simulink model "MBSE_Project_SunRoof"  (R2020b)
settings: Solver=VariableStepAuto  StartTime=0.0  StopTime=inf  RelTol=1e-3
settings Model: Creator=99003747  LastModifiedBy=99003747

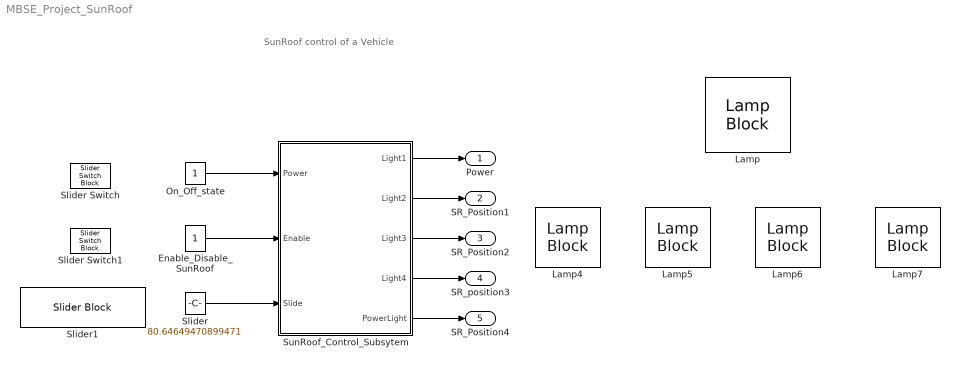
== system MBSE_Project_SunRoof ==
  note: SunRoof control of a Vehicle
  Enable_Disable_SunRoof : Constant
  Lamp{,4..7} (5 alike) : LampBlock
  On_Off_state : Constant
  Slider : Constant  Value=80.64649470899471
  Slider Switch : SliderSwitchBlock
      settings: Values={{'Off', 'On'}, [0 1]}
  Slider Switch1 : SliderSwitchBlock
      settings: Values={{'Off', 'On'}, [0 1]}
  Slider1 : SliderBlock
  SunRoof_Control_Subsytem : Subsystem
      mask Display: image('C:\Users\99003747\Desktop\sunroof.jfif')
  Power : Outport
  SR_Position1 : Outport  Port=2
  SR_Position2 : Outport  Port=3
  SR_position3 : Outport  Port=4
  SR_Position4 : Outport  Port=5
  wires:
  On_Off_state/1 -> SunRoof_Control_Subsytem/1(Power)
  Enable_Disable_SunRoof/1 -> SunRoof_Control_Subsytem/2(Enable)
  Slider/1 -> SunRoof_Control_Subsytem/3(Slide)
  SunRoof_Control_Subsytem/1(Light1) -> Power/1
  SunRoof_Control_Subsytem/2(Light2) -> SR_Position1/1
  SunRoof_Control_Subsytem/3(Light3) -> SR_Position2/1
  SunRoof_Control_Subsytem/4(Light4) -> SR_position3/1
  SunRoof_Control_Subsytem/5(PowerLight) -> SR_Position4/1

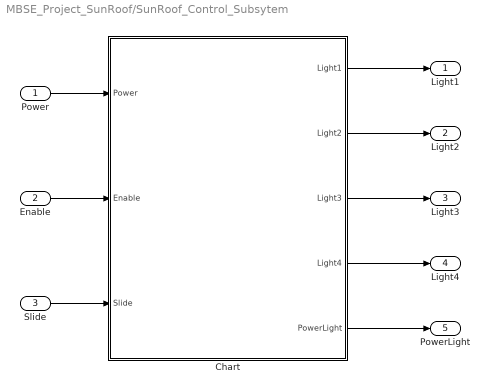
== system MBSE_Project_SunRoof/SunRoof_Control_Subsytem ==
  Power : Inport
  Enable : Inport  Port=2
  Slide : Inport  Port=3
  Chart : Stateflow chart  TreatAsAtomicUnit=on
  Light1 : Outport
  Light2 : Outport  Port=2
  Light3 : Outport  Port=3
  Light4 : Outport  Port=4
  PowerLight : Outport  Port=5
  wires:
  Slide/1 -> Chart/3(Slide)
  Chart/3(Light3) -> Light3/1
  Chart/1(Light1) -> Light1/1
  Chart/2(Light2) -> Light2/1
  Enable/1 -> Chart/2(Enable)
  Power/1 -> Chart/1(Power)
  Chart/4(Light4) -> Light4/1
  Chart/5(PowerLight) -> PowerLight/1

== stateflow chart MBSE_Project_SunRoof/SunRoof_Control_Subsytem/Chart ==
  state PowerOff
    entry:
    PowerLight=0;
    Light1=0;
    Light2=0;
    Light3=0;
    Light4=0;
  state PowerOn
    entry:
    PowerLight=1;
    Light1=0;
    Light2=0;
    Light3=0;
    Light4=0;
  state RoofPosition1
    entry:
    Light1=1;
    Light2=0;
    Light3=0;
    Light4=0;
  state RoofPosition2
    entry:
    Light1=1;
    Light2=1;
    Light3=0;
    Light4=0;
  state RoofPosition4
    entry:
    Light1=1;
    Light2=1;
    Light3=1;
    Light4=1;
  state RoofPosition3
    entry:
    Light1=1;
    Light2=1;
    Light3=1;
    Light4=0;
  (default) -> PowerOff
  PowerOn -> RoofPosition4 [order 2] : [Enable ==1 && Slide>75 && Slide<=100]
  PowerOff -> PowerOn : [Power == 1  ]
  RoofPosition4 -> PowerOn [order 1] : [Enable == 0]
  PowerOn -> PowerOff [order 5] : [Power == 0]
  RoofPosition1 -> PowerOn [order 4] : [Enable ==1 && Slide<=0 && Slide>25]
  PowerOn -> RoofPosition1 [order 4] : [Enable ==1 && Slide>0 && Slide<25]
  RoofPosition1 -> PowerOff [order 2] : [Power == 0]
  RoofPosition1 -> PowerOn [order 1] : [Enable == 0]
  RoofPosition4 -> PowerOff [order 2] : [Power == 0]
  PowerOn -> RoofPosition2 [order 3] : [Enable ==1 && Slide>=25 && Slide<50]
  RoofPosition2 -> PowerOn [order 1] : [Enable == 0]
  RoofPosition3 -> PowerOn [order 1] : [Enable == 0]
  PowerOn -> RoofPosition3 [order 1] : [Enable ==1 && Slide>=50 && Slide<75]
  RoofPosition2 -> PowerOff [order 2] : [Power == 0]
  RoofPosition3 -> PowerOff [order 2] : [Power == 0]
  RoofPosition2 -> RoofPosition1 [order 3] : [Enable ==1 && Slide<=25 && Slide>0]
  RoofPosition3 -> RoofPosition2 [order 3] : [Enable ==1 && Slide<=50 && Slide>25]
  RoofPosition4 -> RoofPosition3 [order 3] : [Enable ==1 && Slide<=75 && Slide>50]
  RoofPosition1 -> RoofPosition2 [order 3] : [Enable ==1 && Slide>=25 && Slide<50]
  RoofPosition2 -> RoofPosition3 [order 4] : [Enable ==1 && Slide>=50 && Slide<75]
  RoofPosition3 -> RoofPosition4 [order 4] : [Enable ==1 && Slide>=75 && Slide<100]
  data: Power input; Light1 output; Enable input; Light2 output; Light3 output; Light4 output; Slide input; PowerLight output
